simulink model "simple"  (R2017b)
settings: Solver=FixedStepDiscrete  StartTime=0.0  StopTime=19.8  FixedStep=0.2  RelTol=1e-3  EnableMultiTasking=on
model workspace (MAT data in the model file):
  already_pp = 1
settings Model: Creator=hbourbou  LastModifiedBy=hbourbou
settings DataIOCC: LimitDataPoints=on  SaveFormat=Structure
settings OptimizationCC: LifeSpan=inf
settings DebuggingCC: AlgebraicLoopMsg=error  SFUnexpectedBacktrackingDiag=warning  SFNoUnconditionalDefaultTransitionDiag=warning  SFExecutionAtInitializationDiag=none
settings HardwareCC: ProdBitPerSizeT=32  ProdBitPerPtrDiffT=32  ProdWordSize=32  ProdHWDeviceType=Specified
settings ModelReferenceCC: PropagateSignalLabelsOutOfModel=off
settings CodeAppCC: StateflowObjectComments=on
settings GRTTargetCC: TargetLangStandard=C89/C90 (ANSI)
settings ConfigComp: CovMetricSettings=dw  CovHtmlReporting=on  CovSaveCumulativeToWorkspaceVar=on  CovSaveSingleToWorkspaceVar=on  CovExternalEMLEnable=off

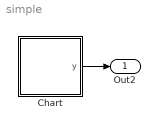
== system simple ==
  Chart : Stateflow chart  TreatAsAtomicUnit=on
  Out2 : Outport
  wires:
  Chart/1(y) -> Out2/1

== stateflow chart simple/Chart ==
  state A
    state B
      en:
      x =  0.0;
      y=0.0;
      du:
      x = x + 1.0;
      y = x -1.0;
    (default) -> B [order 1] : [x==0.0]
    (default) -> B [order 2]
  state C
    du: y = y + 1
  (default) -> A
  B -> C : [x+1.0>y]{x = x - 1.0;}/{y = y+ 1.0;}
  data: y output double; l local double; x local double =0
